simulink model "sim4el17128"  (R2019b)
settings: Solver=VariableStepAuto  StartTime=0.0  StopTime=20  RelTol=1e-4
values from neighbouring files (symbols this model uses):
  b1 = 0.0886    [sim_cm.m]    (also in sim_cm_LM_overestimate.m; sim_cm_LM_underestimate.m; sim_cm_RR_overestimate.m; sim_cm_RR_underestimate.m)
  b2 = 0.0012    [sim_cm.m]    (also in sim_cm_LM_overestimate.m; sim_cm_LM_underestimate.m; sim_cm_RR_overestimate.m; sim_cm_RR_underestimate.m)
  ba = (2*K^2*(alphaS*J-b1))/(3*np^2)    [sim_cm.m]    (also in sim_cm_LM_overestimate.m; sim_cm_LM_underestimate.m; sim_cm_RR_overestimate.m; sim_cm_RR_underestimate.m)
  Idref = psi_hat/LM_hat    (= 4.50282942603)    [sim_cm.m]    (also in sim_cm_LM_overestimate.m = 4.09348129639; sim_cm_LM_underestimate.m = 5.0031438067; sim_cm_RR_overestimate.m; sim_cm_RR_underestimate.m)
  Imax = 12    [sim_cm.m]    (also in sim_cm_LM_overestimate.m; sim_cm_LM_underestimate.m; sim_cm_RR_overestimate.m; sim_cm_RR_underestimate.m = 15)
  Iqref = sqrt(Iref^2-Idref^2)    [sim_cm.m]    (also in sim_cm_LM_overestimate.m; sim_cm_LM_underestimate.m; sim_cm_RR_overestimate.m; sim_cm_RR_underestimate.m)
  J = 0.08    [sim_cm.m]    (also in sim_cm_LM_overestimate.m; sim_cm_LM_underestimate.m; sim_cm_RR_overestimate.m; sim_cm_RR_underestimate.m)
  K = 1/sqrt(2)    [sim_cm.m]    (also in sim_cm_LM_overestimate.m; sim_cm_LM_underestimate.m; sim_cm_RR_overestimate.m; sim_cm_RR_underestimate.m)
  Ki = alphaC*(R+Ra)    [sim_cm.m]    (also in sim_cm_LM_overestimate.m; sim_cm_LM_underestimate.m; sim_cm_RR_overestimate.m; sim_cm_RR_underestimate.m)
  kip = alphaP*alphaP/psi_hat    (= 21723.518851)    [sim_cm.m]    (also in sim_cm_LM_overestimate.m; sim_cm_LM_underestimate.m; sim_cm_RR_overestimate.m; sim_cm_RR_underestimate.m)
  Kis = Kps*alphaS    [sim_cm.m]    (also in sim_cm_LM_overestimate.m; sim_cm_LM_underestimate.m; sim_cm_RR_overestimate.m; sim_cm_RR_underestimate.m)
  Kp = alphaC*L    [sim_cm.m]    (also in sim_cm_LM_overestimate.m; sim_cm_LM_underestimate.m; sim_cm_RR_overestimate.m; sim_cm_RR_underestimate.m)
  kpp = 2*alphaP/psi_hat    (= 394.973070018)    [sim_cm.m]    (also in sim_cm_LM_overestimate.m; sim_cm_LM_underestimate.m; sim_cm_RR_overestimate.m; sim_cm_RR_underestimate.m)
  Kps = (2*K^2*alphaS*J)/(3*np^2)    [sim_cm.m]    (also in sim_cm_LM_overestimate.m; sim_cm_LM_underestimate.m; sim_cm_RR_overestimate.m; sim_cm_RR_underestimate.m)
  L = Lsigma_hat    (= 0.0227)    [sim_cm.m]    (also in sim_cm_LM_overestimate.m; sim_cm_LM_underestimate.m; sim_cm_RR_overestimate.m; sim_cm_RR_underestimate.m)
  lamda = 2    [sim_cm.m]    (also in sim_cm_LM_overestimate.m; sim_cm_LM_underestimate.m; sim_cm_RR_overestimate.m; sim_cm_RR_underestimate.m)
  LM = 0.1237    [sim_cm.m]    (also in sim_cm_LM_overestimate.m; sim_cm_LM_underestimate.m; sim_cm_RR_overestimate.m; sim_cm_RR_underestimate.m)
  LM_hat = LM    (= 0.1237)    [sim_cm.m]    (also in sim_cm_LM_overestimate.m = 0.13607; sim_cm_LM_underestimate.m = 0.11133; sim_cm_RR_overestimate.m; sim_cm_RR_underestimate.m)
  Lsigma = 0.0227    [sim_cm.m]    (also in sim_cm_LM_overestimate.m; sim_cm_LM_underestimate.m; sim_cm_RR_overestimate.m; sim_cm_RR_underestimate.m)
  Lsigma_hat = Lsigma    (= 0.0227)    [sim_cm.m]    (also in sim_cm_LM_overestimate.m; sim_cm_LM_underestimate.m; sim_cm_RR_overestimate.m; sim_cm_RR_underestimate.m)
  np = 2    [sim_cm.m]    (also in sim_cm_LM_overestimate.m; sim_cm_LM_underestimate.m; sim_cm_RR_overestimate.m; sim_cm_RR_underestimate.m)
  phi_a = 0    [sim_cm.m]    (also in sim_cm_LM_overestimate.m; sim_cm_LM_underestimate.m; sim_cm_RR_overestimate.m; sim_cm_RR_underestimate.m)
  phi_b = -2*pi/3    (= -2.09439510239)    [sim_cm.m]    (also in sim_cm_LM_overestimate.m; sim_cm_LM_underestimate.m; sim_cm_RR_overestimate.m; sim_cm_RR_underestimate.m)
  phi_c = -4*pi/3    (= -4.18879020479)    [sim_cm.m]    (also in sim_cm_LM_overestimate.m; sim_cm_LM_underestimate.m; sim_cm_RR_overestimate.m; sim_cm_RR_underestimate.m)
  Ra = alphaC*L - R    [sim_cm.m]    (also in sim_cm_LM_overestimate.m; sim_cm_LM_underestimate.m; sim_cm_RR_overestimate.m; sim_cm_RR_underestimate.m)
  RR = 0.8197    [sim_cm.m]    (also in sim_cm_LM_overestimate.m; sim_cm_LM_underestimate.m; sim_cm_RR_overestimate.m; sim_cm_RR_underestimate.m)
  RR_hat = RR    (= 0.8197)    [sim_cm.m]    (also in sim_cm_LM_overestimate.m; sim_cm_LM_underestimate.m; sim_cm_RR_overestimate.m = 1.14758; sim_cm_RR_underestimate.m = 0.49182)
  Rs = 2.2667    [sim_cm.m]    (also in sim_cm_LM_overestimate.m; sim_cm_LM_underestimate.m; sim_cm_RR_overestimate.m; sim_cm_RR_underestimate.m)
  Rs_hat = Rs    (= 2.2667)    [sim_cm.m]    (also in sim_cm_LM_overestimate.m; sim_cm_LM_underestimate.m; sim_cm_RR_overestimate.m; sim_cm_RR_underestimate.m)
  sw1 = 1    [sim_cm.m]    (also in sim_cm_LM_overestimate.m; sim_cm_LM_underestimate.m; sim_cm_RR_overestimate.m; sim_cm_RR_underestimate.m)
  sw3 = 1    [sim_cm.m]    (also in sim_cm_LM_overestimate.m; sim_cm_LM_underestimate.m; sim_cm_RR_overestimate.m; sim_cm_RR_underestimate.m)
  sw4 = 1    [sim_cm.m]    (also in sim_cm_LM_overestimate.m; sim_cm_LM_underestimate.m; sim_cm_RR_overestimate.m; sim_cm_RR_underestimate.m)
  sw5 = 0    [sim_cm.m]    (also in sim_cm_LM_overestimate.m = 1; sim_cm_LM_underestimate.m = 1; sim_cm_RR_overestimate.m = 1; sim_cm_RR_underestimate.m = 1)
  sw6 = 0    [sim_cm.m]    (also in sim_cm_LM_overestimate.m; sim_cm_LM_underestimate.m; sim_cm_RR_overestimate.m; sim_cm_RR_underestimate.m)
  sw7 = 0    [sim_cm.m]    (also in sim_cm_LM_overestimate.m; sim_cm_LM_underestimate.m; sim_cm_RR_overestimate.m; sim_cm_RR_underestimate.m)
  tL = 26.8    [sim_cm.m]    (also in sim_cm_LM_overestimate.m; sim_cm_LM_underestimate.m; sim_cm_RR_overestimate.m; sim_cm_RR_underestimate.m)
  Un = 230    [sim_cm.m]    (also in sim_cm_LM_overestimate.m; sim_cm_LM_underestimate.m; sim_cm_RR_overestimate.m; sim_cm_RR_underestimate.m)
  Vhat = 230*sqrt(2)    [sim_cm.m]    (also in sim_cm_LM_overestimate.m; sim_cm_LM_underestimate.m; sim_cm_RR_overestimate.m; sim_cm_RR_underestimate.m)
  w = 2*pi*f    (= 314.159265359)    [sim_cm.m]    (also in sim_cm_LM_overestimate.m; sim_cm_LM_underestimate.m; sim_cm_RR_overestimate.m; sim_cm_RR_underestimate.m)
  wdelta = 0.2*wbase    (= 60.48)    [sim_cm.m]    (also in sim_cm_LM_overestimate.m; sim_cm_LM_underestimate.m; sim_cm_RR_overestimate.m; sim_cm_RR_underestimate.m)
undefined symbols (not defined in the file or in its folder): magnitude, sigbuilder_block
libraries: simulink x1
settings Model: DataTypeOverride=Double  MinMaxOverflowLogging=ForceOff  Creator=user  LastModifiedBy=user
settings SolverCC: ZeroCrossAlgorithm=Adaptive
settings DebuggingCC: IgnoredZcDiagnostic=none

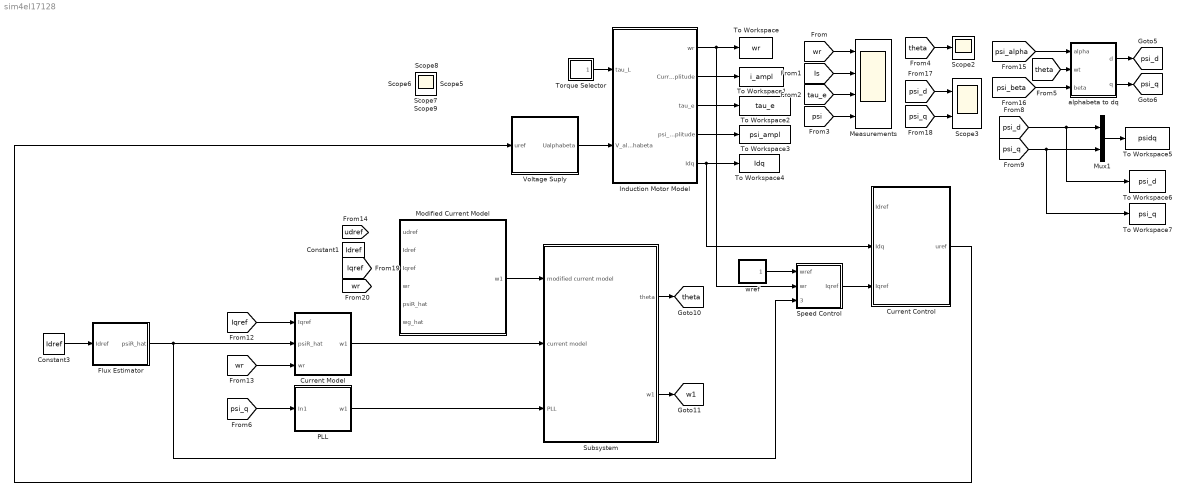
== system sim4el17128 ==
  Constant1 : Constant  Value=Idref
  Constant3 : Constant  Value=Idref
  Current Control : Subsystem
  Current Model : Subsystem
  Flux Estimator : Subsystem
  Induction Motor Model : Subsystem
  Measurements : Scope  NumInputPorts=4
  Modified Current Model : Subsystem
  Mux1 : Mux  Inputs=2
  PLL : Subsystem
  Scope{,1..2,4..9} (9 alike) : Scope
  Scope3 : Scope  NumInputPorts=2
  Speed Control : Subsystem
  Subsystem : Subsystem
  To Workspace : ToWorkspace  VariableName=wr  SaveFormat=Timeseries  SampleTime=-1
  To Workspace1 : ToWorkspace  VariableName=i_ampl  SaveFormat=Timeseries  SampleTime=-1
  To Workspace2 : ToWorkspace  VariableName=tau_e  SaveFormat=Timeseries  SampleTime=-1
  To Workspace3 : ToWorkspace  VariableName=psi_ampl  SaveFormat=Timeseries  SampleTime=-1
  To Workspace4 : ToWorkspace  VariableName=Idq  SaveFormat=Timeseries  SampleTime=-1
  To Workspace5 : ToWorkspace  VariableName=psidq  SaveFormat=Timeseries  SampleTime=-1
  To Workspace6 : ToWorkspace  VariableName=psi_d  SaveFormat=Timeseries  SampleTime=-1
  To Workspace7 : ToWorkspace  VariableName=psi_q  SaveFormat=Timeseries  SampleTime=-1
  Torque Selector : Subsystem
  Voltage Suply : Subsystem
  alphabeta to dq : Subsystem
  wref : Subsystem
  tag scope: psi_d=global, psi_q=global, theta=global, w1=global
  wires:
  Induction Motor Model/1(wr) -> Speed Control/2(wr), To Workspace/1
  Induction Motor Model/3(tau_e) -> To Workspace2/1
  Induction Motor Model/2(Current amplitude) -> To Workspace1/1
  Induction Motor Model/4(psi_amplitude) -> To Workspace3/1
  [wr] -> Measurements/1
  [Is] -> Measurements/2
  [tau_e] -> Measurements/3
  [psi] -> Measurements/4
  [theta] -> Scope2/1
  [psi_q] -> Scope3/2
  [psi_d] -> Scope3/1
  alphabeta to dq/2(q) -> [psi_q]
  [psi_alpha] -> alphabeta to dq/1(alpha)
  [psi_beta] -> alphabeta to dq/3(beta)
  alphabeta to dq/1(d) -> [psi_d]
  Induction Motor Model/5(Idq) -> To Workspace4/1, Current Control/2(Idq)
  Torque Selector/1(tau_L) -> Induction Motor Model/1(tau_L)
  [psi_q] -> To Workspace7/1, Mux1/2
  [psi_d] -> To Workspace6/1, Mux1/1
  Mux1/1 -> To Workspace5/1
  Current Control/1(uref) -> Voltage Suply/1(uref)
  Voltage Suply/1(Ualphabeta) -> Induction Motor Model/2(V_alphabeta)
  Speed Control/1(Iqref) -> Current Control/3(Iqref)
  wref/1(Out1) -> Speed Control/1(wref)
  [theta] -> alphabeta to dq/2(wt)
  Subsystem/1(theta) -> [theta]
  Subsystem/2(w1) -> [w1]
  [Iqref] -> Current Model/1(Iqref)
  [wr] -> Current Model/3(wr)
  [psi_q] -> PLL/1(In1)
  Current Model/1(w1) -> Subsystem/2(current model)
  PLL/1(w1) -> Subsystem/3(PLL)
  Constant3/1 -> Flux Estimator/1(Idref)
  Flux Estimator/1(psiR_hat) -> Speed Control/3(psiR_hat), Current Model/2(psiR_hat)
  Modified Current Model/1(w1) -> Subsystem/1(modified current model)

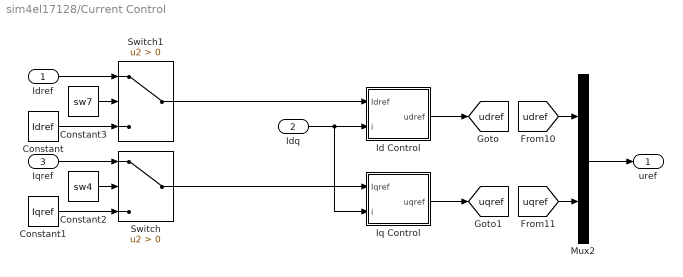
== system sim4el17128/Current Control ==
  Idref : Inport
  Idq : Inport  Port=2
  Iqref : Inport  Port=3
  Constant : Constant  Value=Idref
  Constant1 : Constant  Value=Iqref
  Constant2 : Constant  Value=sw4
  Constant3 : Constant  Value=sw7
  Id Control : Subsystem
  Iq Control : Subsystem
  Mux2 : Mux  Inputs=2
  Switch : Switch  Criteria=u2 > Threshold
  Switch1 : Switch  Criteria=u2 > Threshold
  uref : Outport
  tag scope: udref=global, uqref=global
  wires:
  [uqref] -> Mux2/2
  Iq Control/1(uqref) -> [uqref]
  Idq/1 -> Id Control/2(i), Iq Control/2(i)
  Mux2/1 -> uref/1
  [udref] -> Mux2/1
  Id Control/1(udref) -> [udref]
  Iqref/1 -> Switch/1
  Switch/1 -> Iq Control/1(Iqref)
  Constant2/1 -> Switch/2
  Constant1/1 -> Switch/3
  Switch1/1 -> Id Control/1(Idref)
  Constant/1 -> Switch1/3
  Constant3/1 -> Switch1/2
  Idref/1 -> Switch1/1

== system sim4el17128/Current Model ==
  Iqref : Inport
  psiR_hat : Inport  Port=2
  wr : Inport  Port=3
  Gain : Gain  Gain=RR_hat
  Product : Product  Inputs=*/
  Sum : Sum
  w1 : Outport
  wires:
  wr/1 -> Sum/2
  Sum/1 -> w1/1
  Iqref/1 -> Gain/1
  Gain/1 -> Product/1
  Product/1 -> Sum/1
  psiR_hat/1 -> Product/2

== system sim4el17128/Flux Estimator ==
  Idref : Inport
  Clock : Clock
  Constant4 : Constant  Value=0.001
  Gain : Gain  Gain=RR_hat
  Gain1 : Gain  Gain=1/LM_hat
  Integrator : Integrator
  Sum : Sum  Inputs=|+-
  Switch : Switch  Criteria=u2 > Threshold  Threshold=0.001
  psiR_hat : Outport
  wires:
  Clock/1 -> Switch/2
  Constant4/1 -> Switch/3
  Integrator/1 -> Gain1/1, Switch/1
  Gain1/1 -> Sum/2
  Sum/1 -> Gain/1
  Gain/1 -> Integrator/1
  Idref/1 -> Sum/1
  Switch/1 -> psiR_hat/1

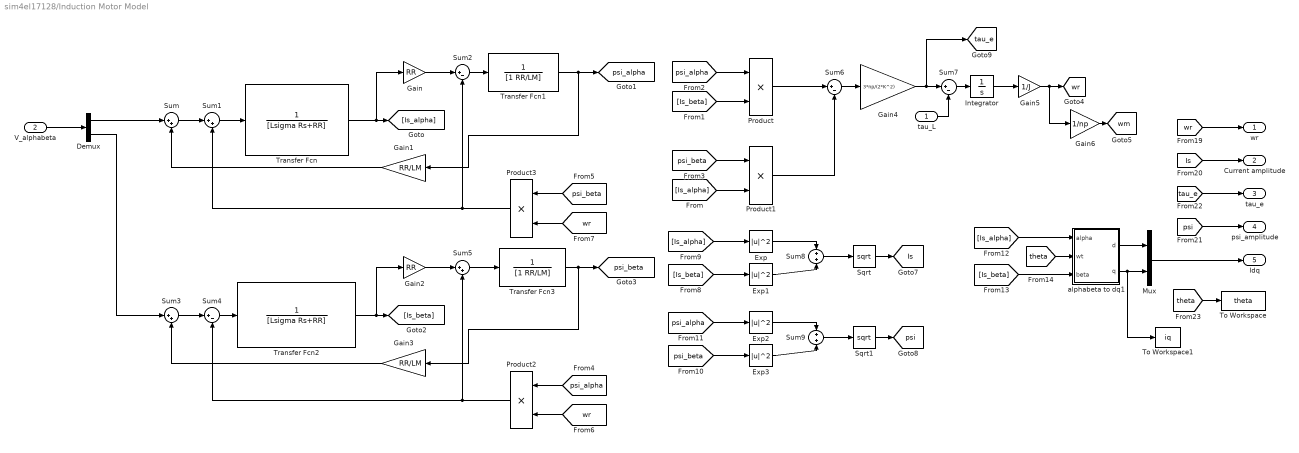
== system sim4el17128/Induction Motor Model ==
  tau_L : Inport
  V_alphabeta : Inport  Port=2
  Demux : Demux  Outputs=2
  Exp{,1..3} (4 alike) : Math  Operator=magnitude^2  SignedPower=off  SaturateOnIntegerOverflow=on
  Gain : Gain  Gain=RR
  Gain1 : Gain  Gain=RR/LM
  Gain2 : Gain  Gain=RR
  Gain3 : Gain  Gain=RR/LM
  Gain4 : Gain  Gain=3*np/(2*K^2)
  Gain5 : Gain  Gain=1/J
  Gain6 : Gain  Gain=1/np
  Integrator : Integrator
  Mux : Mux  Inputs=2
  Product{,1..3} (4 alike) : Product
  Sqrt : Sqrt  SaturateOnIntegerOverflow=on
  Sqrt1 : Sqrt  SaturateOnIntegerOverflow=on
  Sum{,1,3,5} (4 alike) : Sum  Inputs=|++
  Sum{2,4,6..7} (4 alike) : Sum  Inputs=|+-
  Sum8 : Sum  Inputs=+|+
  Sum9 : Sum  Inputs=+|+
  To Workspace : ToWorkspace  VariableName=theta  SaveFormat=Timeseries  SampleTime=-1
  To Workspace1 : ToWorkspace  VariableName=iq  SaveFormat=Timeseries  SampleTime=-1
  Transfer Fcn : TransferFcn  Denominator=[Lsigma Rs+RR]
  Transfer Fcn1 : TransferFcn  Denominator=[1 RR/LM]
  Transfer Fcn2 : TransferFcn  Denominator=[Lsigma Rs+RR]
  Transfer Fcn3 : TransferFcn  Denominator=[1 RR/LM]
  alphabeta to dq1 : Subsystem
  wr : Outport
  Current amplitude : Outport  Port=2
  tau_e : Outport  Port=3
  psi_amplitude : Outport  Port=4
  Idq : Outport  Port=5
  tag scope: Is=global, psi=global, psi_alpha=global, psi_beta=global, tau_e=global, wm=global, wr=global
  wires:
  Transfer Fcn1/1 -> Gain1/1, [psi_alpha]
  Product3/1 -> Sum1/2, Sum2/2
  Product2/1 -> Sum4/2, Sum5/2
  [Is_beta] -> Exp1/1
  Gain5/1 -> Gain6/1, [wr]
  [Is_beta] -> Product/2
  Product/1 -> Sum6/1
  [wr] -> Product2/2
  Sqrt/1 -> [Is]
  Sum3/1 -> Sum4/1
  Transfer Fcn3/1 -> Gain3/1, [psi_beta]
  [psi_beta] -> Product1/1
  Sum5/1 -> Transfer Fcn3/1
  Transfer Fcn2/1 -> Gain2/1, [Is_beta]
  Sum1/1 -> Transfer Fcn/1
  V_alphabeta/1 -> Demux/1
  [Is_alpha] -> Product1/2
  Gain1/1 -> Sum/2
  Demux/2 -> Sum3/1
  Demux/1 -> Sum/1
  Exp/1 -> Sum8/1
  tau_L/1 -> Sum7/2
  Sum/1 -> Sum1/1
  Sum6/1 -> Gain4/1
  Gain4/1 -> [tau_e], Sum7/1
  Transfer Fcn/1 -> Gain/1, [Is_alpha]
  [psi_alpha] -> Product/1
  Sum2/1 -> Transfer Fcn1/1
  Gain3/1 -> Sum3/2
  Gain2/1 -> Sum5/1
  Sum4/1 -> Transfer Fcn2/1
  Product1/1 -> Sum6/2
  [Is_alpha] -> Exp/1
  Sum8/1 -> Sqrt/1
  Gain/1 -> Sum2/1
  [wr] -> Product3/2
  [psi_beta] -> Product3/1
  Sum7/1 -> Integrator/1
  Integrator/1 -> Gain5/1
  [psi_alpha] -> Product2/1
  Exp1/1 -> Sum8/2
  Sum9/1 -> Sqrt1/1
  [psi_alpha] -> Exp2/1
  Exp3/1 -> Sum9/2
  [psi_beta] -> Exp3/1
  Exp2/1 -> Sum9/1
  Sqrt1/1 -> [psi]
  Mux/1 -> Idq/1
  alphabeta to dq1/2(q) -> To Workspace1/1, Mux/2
  alphabeta to dq1/1(d) -> Mux/1
  [Is_beta] -> alphabeta to dq1/3(beta)
  [Is_alpha] -> alphabeta to dq1/1(alpha)
  [theta] -> alphabeta to dq1/2(wt)
  [wr] -> wr/1
  [Is] -> Current amplitude/1
  [psi] -> psi_amplitude/1
  [tau_e] -> tau_e/1
  [theta] -> To Workspace/1
  Gain6/1 -> [wm]

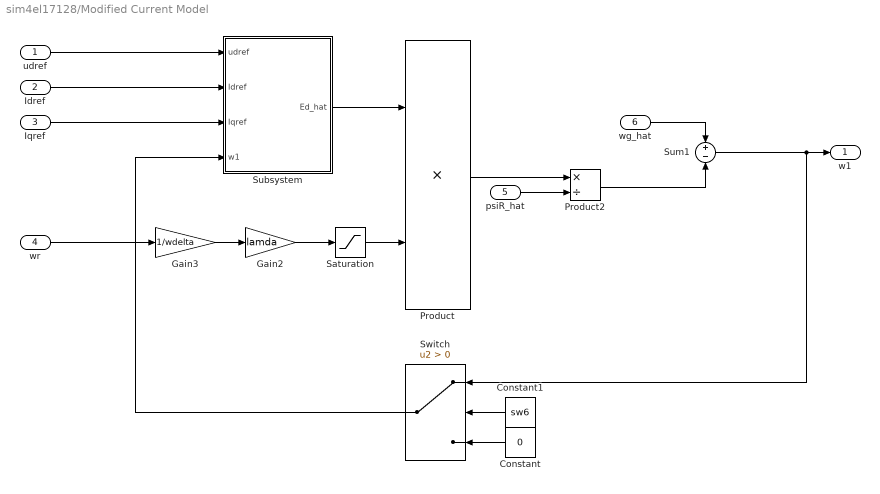
== system sim4el17128/Modified Current Model ==
  udref : Inport
  Idref : Inport  Port=2
  Iqref : Inport  Port=3
  wr : Inport  Port=4
  psiR_hat : Inport  Port=5
  wg_hat : Inport  Port=6
  Constant : Constant  Value=0
  Constant1 : Constant  Value=sw6
  Gain2 : Gain  Gain=lamda
  Gain3 : Gain  Gain=1/wdelta
  Product : Product
  Product2 : Product  Inputs=*/
  Saturation : Saturate  UpperLimit=lamda  LowerLimit=-lamda
  Subsystem : Subsystem
  Sum1 : Sum  Inputs=+-
  Switch : Switch  Criteria=u2 > Threshold
  w1 : Outport
  wires:
  Sum1/1 -> Switch/1, w1/1
  Product/1 -> Product2/1
  Switch/1 -> Subsystem/4(w1)
  Constant/1 -> Switch/3
  Constant1/1 -> Switch/2
  Idref/1 -> Subsystem/2(Idref)
  udref/1 -> Subsystem/1(udref)
  Subsystem/1(Ed_hat) -> Product/1
  Gain3/1 -> Gain2/1
  Gain2/1 -> Saturation/1
  Saturation/1 -> Product/2
  Iqref/1 -> Subsystem/3(Iqref)
  wr/1 -> Gain3/1
  psiR_hat/1 -> Product2/2
  Product2/1 -> Sum1/2
  wg_hat/1 -> Sum1/1

== system sim4el17128/PLL ==
  In1 : Inport
  Gain8 : Gain  Gain=kpp
  Gain9 : Gain  Gain=kip
  Integrator1 : Integrator
  Sum13 : Sum  Inputs=+++
  wg : Constant  Value=w
  w1 : Outport
  wires:
  In1/1 -> Gain9/1, Gain8/1  "ψq"
  Gain8/1 -> Sum13/2
  wg/1 -> Sum13/1
  Gain9/1 -> Integrator1/1
  Integrator1/1 -> Sum13/3
  Sum13/1 -> w1/1

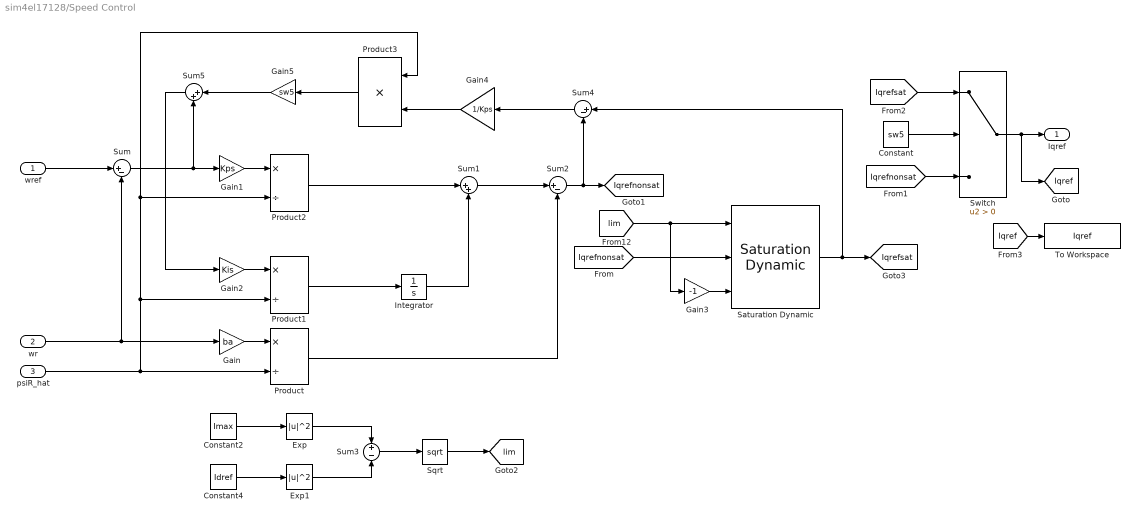
== system sim4el17128/Speed Control ==
  wref : Inport
  wr : Inport  Port=2
  psiR_hat : Inport  Port=3
  Constant : Constant  Value=sw5
  Constant2 : Constant  Value=Imax
  Constant4 : Constant  Value=Idref
  Exp : Math  Operator=magnitude^2  SignedPower=off  SaturateOnIntegerOverflow=on
  Exp1 : Math  Operator=magnitude^2  SignedPower=off  SaturateOnIntegerOverflow=on
  Gain : Gain  Gain=ba
  Gain1 : Gain  Gain=Kps
  Gain2 : Gain  Gain=Kis
  Gain3 : Gain  Gain=-1
  Gain4 : Gain  Gain=1/Kps
  Gain5 : Gain  Gain=sw5
  Integrator : Integrator
  Product : Product  Inputs=*/
  Product1 : Product  Inputs=*/
  Product2 : Product  Inputs=*/
  Product3 : Product
  Saturation Dynamic : simulink/Discontinuities/Saturation Dynamic  OutMin=[]  OutMax=[]  OutDataTypeStr=Inherit: Same as second input  OutDataType=fixdt(1, 16)  OutScaling=2^-10  DoSatur=off
  Sqrt : Sqrt  SaturateOnIntegerOverflow=on
  Sum : Sum  Inputs=|+-
  Sum1 : Sum  Inputs=|++
  Sum2 : Sum  Inputs=|+-
  Sum3 : Sum  Inputs=+-
  Sum4 : Sum  Inputs=|+-
  Sum5 : Sum  Inputs=|++
  Switch : Switch  Criteria=u2 > Threshold
  To Workspace : ToWorkspace  VariableName=Iqref  SaveFormat=Timeseries  SampleTime=-1
  Iqref : Outport
  tag scope: Iqref=global, Iqrefnonsat=global, Iqrefsat=global, lim=global
  wires:
  Sum3/1 -> Sqrt/1
  Exp/1 -> Sum3/1
  Sum/1 -> Sum5/2, Gain1/1
  Gain3/1 -> Saturation Dynamic/3
  wr/1 -> Sum/2, Gain/1
  Constant4/1 -> Exp1/1
  Exp1/1 -> Sum3/2
  Sum1/1 -> Sum2/1
  Sum4/1 -> Gain4/1
  Integrator/1 -> Sum1/2
  wref/1 -> Sum/1
  Gain5/1 -> Sum5/1
  [lim] -> Gain3/1, Saturation Dynamic/1
  Sum2/1 -> Sum4/2, [Iqrefnonsat]
  [Iqrefnonsat] -> Saturation Dynamic/2
  Saturation Dynamic/1 -> [Iqrefsat], Sum4/1
  [Iqrefnonsat] -> Switch/3
  Switch/1 -> Iqref/1, [Iqref]
  [Iqrefsat] -> Switch/1
  Constant/1 -> Switch/2
  Sum5/1 -> Gain2/1
  Sqrt/1 -> [lim]
  Gain/1 -> Product/1
  Product/1 -> Sum2/2
  Constant2/1 -> Exp/1
  psiR_hat/1 -> Product/2, Product1/2, Product2/2, Product3/1
  Gain2/1 -> Product1/1
  Product1/1 -> Integrator/1
  Gain1/1 -> Product2/1
  Product2/1 -> Sum1/1
  Product3/1 -> Gain5/1
  Gain4/1 -> Product3/2
  [Iqref] -> To Workspace/1

== system sim4el17128/Subsystem ==
  modified current model : Inport
  current model : Inport  Port=2
  PLL : Inport  Port=3
  Constant : Constant  Value=sw4
  Constant1 : Constant  Value=sw6
  Constant2 : Constant  Value=sw7
  Constant5 : Constant  Value=2*pi
  Integrator2 : Integrator
  Mod : Math  Operator=mod  SignedPower=off  SaturateOnIntegerOverflow=on
  Switch : Switch  Criteria=u2 > Threshold
  Switch1 : Switch  Criteria=u2 > Threshold
  Switch2 : Switch  Criteria=u2 > Threshold
  theta : Outport
  w1 : Outport  Port=2
  wires:
  modified current model/1 -> Switch1/1
  Constant/1 -> Switch/2
  Constant1/1 -> Switch1/2
  Switch/1 -> Switch1/3
  current model/1 -> Switch/1
  PLL/1 -> Switch/3
  Mod/1 -> theta/1
  Constant5/1 -> Mod/2
  Integrator2/1 -> Mod/1
  Switch1/1 -> Switch2/3
  Switch2/1 -> w1/1, Integrator2/1
  Constant2/1 -> Switch2/2

== system sim4el17128/Torque Selector ==
  Constant : Constant  Value=0
  Exp : Math  Operator=magnitude^2  SignedPower=off  SaturateOnIntegerOverflow=on
  Gain : Gain  Gain=b1
  Gain1 : Gain  Gain=b2
  Manual Switch : ManualSwitch  CurrentSetting=0
  Manual Switch1 : ManualSwitch
  Manual Switch2 : ManualSwitch  CurrentSetting=0
  taul_L : Step  Time=5  After=tL  SampleTime=0
  tau_L : Outport
  wires:
  [wr] -> Gain/1
  Gain1/1 -> Manual Switch1/2
  taul_L/1 -> Manual Switch/2
  Exp/1 -> Gain1/1
  [wm] -> Exp/1
  Constant/1 -> Manual Switch/1
  Gain/1 -> Manual Switch1/1
  Manual Switch2/1 -> tau_L/1
  Manual Switch1/1 -> Manual Switch2/2
  Manual Switch/1 -> Manual Switch2/1

== system sim4el17128/Voltage Suply ==
  uref : Inport
  Constant2 : Constant  Value=sw1
  Demux : Demux  Outputs=2
  Grid Voltage : Subsystem
  Mux : Mux  Inputs=2
  Scope1 : Scope
  Switch : Switch  Criteria=u2 > Threshold
  dq to alphabeta : Subsystem
  Ualphabeta : Outport
  wires:
  Grid Voltage/2(V_dq) -> Scope1/1
  Constant2/1 -> Switch/2
  Mux/1 -> Switch/1
  Demux/2 -> dq to alphabeta/3(q)
  Demux/1 -> dq to alphabeta/1(d)
  Grid Voltage/1(V_alphabeta) -> Switch/3
  [theta] -> dq to alphabeta/2(wt)
  dq to alphabeta/1(alpha) -> Mux/1
  dq to alphabeta/2(beta) -> Mux/2
  uref/1 -> Demux/1
  Switch/1 -> Ualphabeta/1  "Ualphabeta"

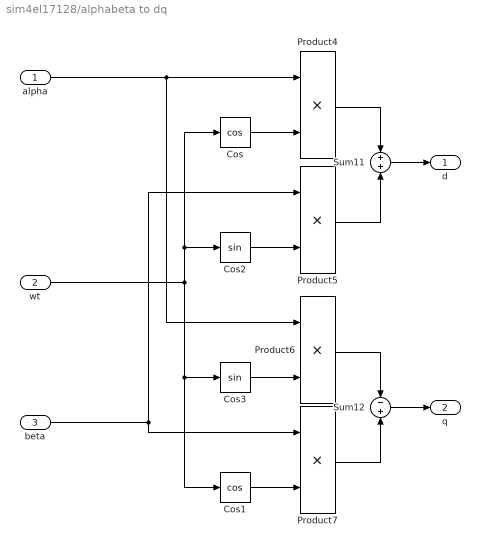
== system sim4el17128/alphabeta to dq ==
  alpha : Inport
  wt : Inport  Port=2
  beta : Inport  Port=3
  Cos : Trigonometry  Operator=cos
  Cos1 : Trigonometry  Operator=cos
  Cos2 : Trigonometry
  Cos3 : Trigonometry
  Product{4..7} (4 alike) : Product
  Sum11 : Sum
  Sum12 : Sum  Inputs=-+
  d : Outport
  q : Outport  Port=2
  wires:
  Cos3/1 -> Product6/2
  Product6/1 -> Sum12/1
  Sum11/1 -> d/1
  alpha/1 -> Product4/1, Product6/1
  wt/1 -> Cos3/1, Cos1/1, Cos2/1, Cos/1
  Product4/1 -> Sum11/1
  beta/1 -> Product7/1, Product5/1
  Product7/1 -> Sum12/2
  Cos1/1 -> Product7/2
  Product5/1 -> Sum11/2
  Cos/1 -> Product4/2
  Cos2/1 -> Product5/2
  Sum12/1 -> q/1

== system sim4el17128/wref ==
  Constant : Constant  Value=sw7
  Manual Switch : ManualSwitch
  Signal Builder : Subsystem  Tag=STV Subsys  LoadFcn=sigbuilder_block('load');  StartFcn=sigbuilder_block('start');  StopFcn=sigbuilder_block('stop');  ClipboardFcn=sigbuilder_block('clipboard');  mask(Sigbuilder block){tuvar=[0:10]}
      mask help: Simulink:masks:SigbuilderBlock_MD
      mask init:
      | if ~strcmp(get_param(bdroot(gcbh),'SimulationStatus'),'stopped') tuvar = sigbuilder_block('maskInit'); end
      settings: CopyFcn=sigbuilder_block('copy');  DeleteFcn=sigbuilder_block('delete');  ModelCloseFcn=sigbuilder_block('modelClose');  PreSaveFcn=sigbuilder_block('preSave');  PauseFcn=sigbuilder_block('pause');  ContinueFcn=sigbuilder_block('continue');  NameChangeFcn=sigbuilder_block('namechange');  OpenFcn=sigbuilder_block('open',[6 30 1012.5 447.75 ]);  CloseFcn=sigbuilder_block('close');
      mask Display: plot(0, 0, 100, 100,[2, 2, 32, 32, 2], [68, 8, 8, 68, 68],[32, 2], [38, 38], [32, 19, 2],[53, 60, 44], [32, 17, 17, 2],[16, 16, 31, 31]);txt = getActiveGroup(gcbh);text(2, 100, txt,'verticalAlignment', 'top');
  Switch : Switch  Criteria=u2 > Threshold
  To Workspace : ToWorkspace  VariableName=wref  SaveFormat=Timeseries  SampleTime=-1
  Out1 : Outport
  wires:
  Signal Builder/2(wrefnom) -> Manual Switch/2
  Signal Builder/1(wref) -> Manual Switch/1
  Manual Switch/1 -> Switch/3
  Signal Builder/3(field weakening) -> Switch/1
  Switch/1 -> To Workspace/1, Out1/1
  Constant/1 -> Switch/2

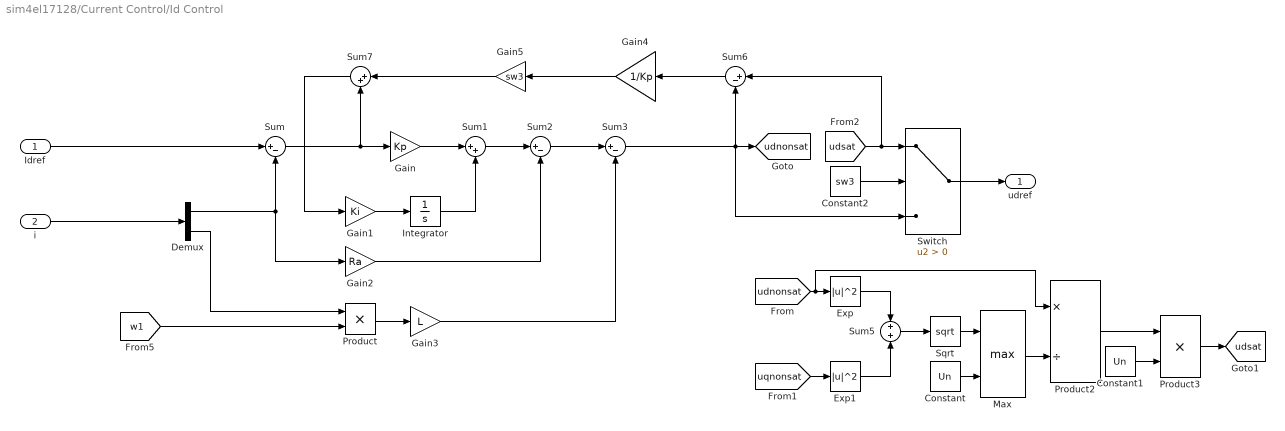
== system sim4el17128/Current Control/Id Control ==
  Idref : Inport
  i : Inport  Port=2
  Constant : Constant  Value=Un
  Constant1 : Constant  Value=Un
  Constant2 : Constant  Value=sw3
  Demux : Demux  Outputs=2
  Exp : Math  Operator=magnitude^2  SignedPower=off  SaturateOnIntegerOverflow=on
  Exp1 : Math  Operator=magnitude^2  SignedPower=off  SaturateOnIntegerOverflow=on
  Gain : Gain  Gain=Kp
  Gain1 : Gain  Gain=Ki
  Gain2 : Gain  Gain=Ra
  Gain3 : Gain  Gain=L
  Gain4 : Gain  Gain=1/Kp
  Gain5 : Gain  Gain=sw3
  Integrator : Integrator
  Max : MinMax  Function=max  Inputs=2
  Product : Product
  Product2 : Product  Inputs=*/
  Product3 : Product
  Sqrt : Sqrt  SaturateOnIntegerOverflow=on
  Sum{,2..3,6} (4 alike) : Sum  Inputs=|+-
  Sum1 : Sum  Inputs=|++
  Sum5 : Sum
  Sum7 : Sum  Inputs=|++
  Switch : Switch  Criteria=u2 > Threshold
  udref : Outport
  tag scope: udnonsat=global, udsat=global
  wires:
  Sum/1 -> Sum7/2, Gain/1
  Demux/2 -> Product/1
  Gain2/1 -> Sum2/2
  Demux/1 -> Gain2/1, Sum/2
  Gain/1 -> Sum1/1
  Sum2/1 -> Sum3/1
  Sum1/1 -> Sum2/1
  Gain1/1 -> Integrator/1
  Product/1 -> Gain3/1
  Integrator/1 -> Sum1/2
  i/1 -> Demux/1
  Idref/1 -> Sum/1
  [udnonsat] -> Product2/1, Exp/1
  [uqnonsat] -> Exp1/1
  Exp/1 -> Sum5/1
  Exp1/1 -> Sum5/2
  Sum5/1 -> Sqrt/1
  Sqrt/1 -> Max/1
  Constant/1 -> Max/2
  Max/1 -> Product2/2
  Product2/1 -> Product3/1
  Constant1/1 -> Product3/2
  Product3/1 -> [udsat]
  [udsat] -> Switch/1, Sum6/1
  Sum7/1 -> Gain1/1
  Gain4/1 -> Gain5/1
  Sum6/1 -> Gain4/1
  [w1] -> Product/2
  Switch/1 -> udref/1
  Constant2/1 -> Switch/2
  Gain5/1 -> Sum7/1
  Gain3/1 -> Sum3/2
  Sum3/1 -> Switch/3, Sum6/2, [udnonsat]

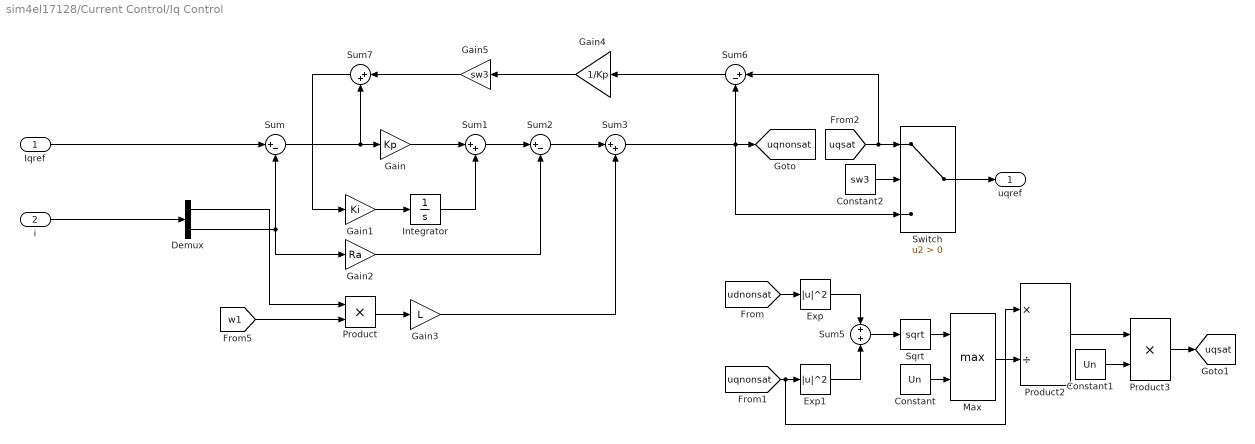
== system sim4el17128/Current Control/Iq Control ==
  Iqref : Inport
  i : Inport  Port=2
  Constant : Constant  Value=Un
  Constant1 : Constant  Value=Un
  Constant2 : Constant  Value=sw3
  Demux : Demux  Outputs=2
  Exp : Math  Operator=magnitude^2  SignedPower=off  SaturateOnIntegerOverflow=on
  Exp1 : Math  Operator=magnitude^2  SignedPower=off  SaturateOnIntegerOverflow=on
  Gain : Gain  Gain=Kp
  Gain1 : Gain  Gain=Ki
  Gain2 : Gain  Gain=Ra
  Gain3 : Gain  Gain=L
  Gain4 : Gain  Gain=1/Kp
  Gain5 : Gain  Gain=sw3
  Integrator : Integrator
  Max : MinMax  Function=max  Inputs=2
  Product : Product
  Product2 : Product  Inputs=*/
  Product3 : Product
  Sqrt : Sqrt  SaturateOnIntegerOverflow=on
  Sum : Sum  Inputs=|+-
  Sum1 : Sum  Inputs=|++
  Sum2 : Sum  Inputs=|+-
  Sum3 : Sum  Inputs=|++
  Sum5 : Sum
  Sum6 : Sum  Inputs=|+-
  Sum7 : Sum  Inputs=|++
  Switch : Switch  Criteria=u2 > Threshold
  uqref : Outport
  tag scope: uqnonsat=global, uqsat=global
  wires:
  Iqref/1 -> Sum/1
  i/1 -> Demux/1
  Integrator/1 -> Sum1/2
  Product/1 -> Gain3/1
  Gain1/1 -> Integrator/1
  Sum1/1 -> Sum2/1
  Sum2/1 -> Sum3/1
  Gain/1 -> Sum1/1
  Gain2/1 -> Sum2/2
  [w1] -> Product/2
  Demux/2 -> Sum/2, Gain2/1
  Demux/1 -> Product/1
  Sum/1 -> Sum7/2, Gain/1
  Exp1/1 -> Sum5/2
  Constant1/1 -> Product3/2
  Max/1 -> Product2/2
  Sum5/1 -> Sqrt/1
  Constant/1 -> Max/2
  Product3/1 -> [uqsat]
  Sqrt/1 -> Max/1
  Product2/1 -> Product3/1
  [uqnonsat] -> Product2/1, Exp1/1
  Exp/1 -> Sum5/1
  [udnonsat] -> Exp/1
  Sum6/1 -> Gain4/1
  Gain4/1 -> Gain5/1
  Sum7/1 -> Gain1/1
  [uqsat] -> Sum6/1, Switch/1
  Switch/1 -> uqref/1
  Constant2/1 -> Switch/2
  Gain5/1 -> Sum7/1
  Sum3/1 -> Switch/3, Sum6/2, [uqnonsat]
  Gain3/1 -> Sum3/2

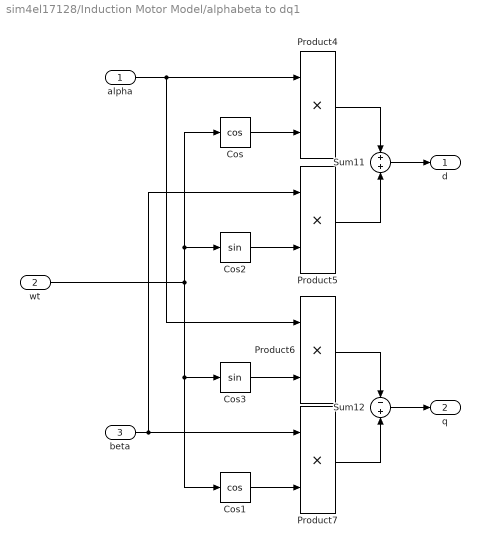
== system sim4el17128/Induction Motor Model/alphabeta to dq1 ==
  alpha : Inport
  wt : Inport  Port=2
  beta : Inport  Port=3
  Cos : Trigonometry  Operator=cos
  Cos1 : Trigonometry  Operator=cos
  Cos2 : Trigonometry
  Cos3 : Trigonometry
  Product{4..7} (4 alike) : Product
  Sum11 : Sum
  Sum12 : Sum  Inputs=-+
  d : Outport
  q : Outport  Port=2
  wires:
  Sum12/1 -> q/1
  Cos2/1 -> Product5/2
  Cos/1 -> Product4/2
  Product5/1 -> Sum11/2
  Cos1/1 -> Product7/2
  Product7/1 -> Sum12/2
  beta/1 -> Product7/1, Product5/1
  Product4/1 -> Sum11/1
  wt/1 -> Cos/1, Cos2/1, Cos1/1, Cos3/1
  alpha/1 -> Product6/1, Product4/1
  Sum11/1 -> d/1
  Product6/1 -> Sum12/1
  Cos3/1 -> Product6/2

== system sim4el17128/Modified Current Model/Subsystem ==
  udref : Inport
  Idref : Inport  Port=2
  Iqref : Inport  Port=3
  w1 : Inport  Port=4
  Gain : Gain  Gain=Rs_hat
  Gain1 : Gain  Gain=Lsigma_hat
  Product : Product
  Sum : Sum  Inputs=+-+
  Ed_hat : Outport
  wires:
  Sum/1 -> Ed_hat/1
  Iqref/1 -> Product/1
  udref/1 -> Sum/1
  Gain/1 -> Sum/2
  Idref/1 -> Gain/1
  Product/1 -> Gain1/1
  Gain1/1 -> Sum/3
  w1/1 -> Product/2

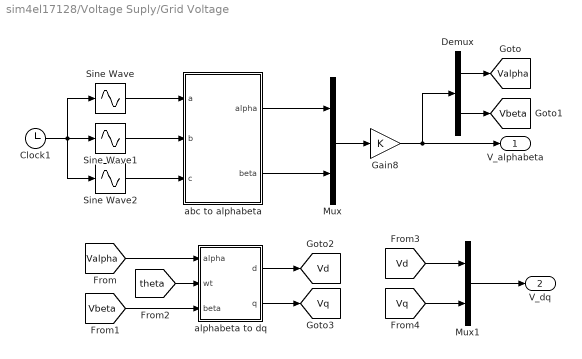
== system sim4el17128/Voltage Suply/Grid Voltage ==
  Clock1 : Clock
  Demux : Demux  Outputs=2
  Gain8 : Gain  Gain=K
  Mux : Mux  Inputs=2
  Mux1 : Mux  Inputs=2
  Sine Wave : Sin  TimeSource=Use external signal  Amplitude=Vhat  Frequency=w  Phase=phi_a  SampleTime=0
  Sine Wave1 : Sin  TimeSource=Use external signal  Amplitude=Vhat  Frequency=w  Phase=phi_b  SampleTime=0
  Sine Wave2 : Sin  TimeSource=Use external signal  Amplitude=Vhat  Frequency=w  Phase=phi_c  SampleTime=0
  abc to alphabeta : Subsystem
  alphabeta to dq : Subsystem
  V_alphabeta : Outport
  V_dq : Outport  Port=2
  tag scope: Valpha=global, Vbeta=global, Vd=global, Vq=global
  wires:
  Clock1/1 -> Sine Wave1/1, Sine Wave2/1, Sine Wave/1
  Mux/1 -> Gain8/1
  Gain8/1 -> Demux/1, V_alphabeta/1
  Demux/2 -> [Vbeta]
  Demux/1 -> [Valpha]
  [Valpha] -> alphabeta to dq/1(alpha)
  [Vbeta] -> alphabeta to dq/3(beta)
  [theta] -> alphabeta to dq/2(wt)
  alphabeta to dq/1(d) -> [Vd]
  alphabeta to dq/2(q) -> [Vq]
  [Vq] -> Mux1/2
  [Vd] -> Mux1/1
  Mux1/1 -> V_dq/1
  Sine Wave/1 -> abc to alphabeta/1(a)
  Sine Wave1/1 -> abc to alphabeta/2(b)
  Sine Wave2/1 -> abc to alphabeta/3(c)
  abc to alphabeta/1(alpha) -> Mux/1
  abc to alphabeta/2(beta) -> Mux/2

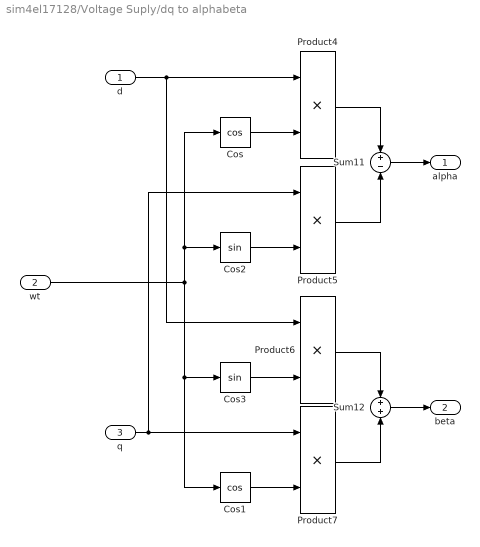
== system sim4el17128/Voltage Suply/dq to alphabeta ==
  d : Inport
  wt : Inport  Port=2
  q : Inport  Port=3
  Cos : Trigonometry  Operator=cos
  Cos1 : Trigonometry  Operator=cos
  Cos2 : Trigonometry
  Cos3 : Trigonometry
  Product{4..7} (4 alike) : Product
  Sum11 : Sum  Inputs=+-
  Sum12 : Sum
  alpha : Outport
  beta : Outport  Port=2
  wires:
  Cos3/1 -> Product6/2
  Product6/1 -> Sum12/1
  Sum11/1 -> alpha/1
  d/1 -> Product4/1, Product6/1
  wt/1 -> Cos3/1, Cos1/1, Cos2/1, Cos/1
  Product4/1 -> Sum11/1
  q/1 -> Product5/1, Product7/1
  Product7/1 -> Sum12/2
  Cos1/1 -> Product7/2
  Product5/1 -> Sum11/2
  Cos/1 -> Product4/2
  Cos2/1 -> Product5/2
  Sum12/1 -> beta/1

== system sim4el17128/wref/Signal Builder ==
  Demux : Demux  Tag=STV Demux  Outputs=3
  FromWs : FromWorkspace  Tag=STV FromWs  VariableName=tuvar  SampleTime=0
      SigBuilderData=|
      | common.afterFinalStr = 'Extrapolate'
      | common.sampleTime = 0
      | dataSet.timeRange = [0 25]
      | dataSet.name = 'Step wref'
      | sbobj.Groups.Name = 'Step wref'
      | sbobj.Groups.Signals(1).Name = 'wref'
      | sbobj.Groups.Signals(1).XData = [0 7 7 20 20 25]
      | sbobj.Groups.Signals(1).YData = [150 150 302.4 302.4 100 100]
      | sbobj.Groups.Signals(2).Name = 'wrefnom'
      | sbobj.Groups.Signals(2).XData = [0 25]
      | sbobj.Groups.Signals(2).YData = [150 150]
      | sbobj.Groups.Signals(3).Name = 'field weakening'
      | sbobj.Groups.Signals(3).XData = [0 25]
      | sbobj.Groups.Signals(3).YData = [1209.6 1209.6]
      | sbobj.Groups.TimeRange = [0 25]
  wref : Outport  Tag=STV Outport
  wrefnom : Outport  Tag=STV Outport  Port=2
  field weakening : Outport  Tag=STV Outport  Port=3
  wires:
  Demux/1 -> wref/1
  FromWs/1 -> Demux/1
  Demux/2 -> wrefnom/1
  Demux/3 -> field weakening/1

== system sim4el17128/Voltage Suply/Grid Voltage/abc to alphabeta ==
  a : Inport
  b : Inport  Port=2
  c : Inport  Port=3
  Gain2 : Gain  Gain=2/3
  Gain3 : Gain  Gain=1/3
  Gain4 : Gain  Gain=1/3
  Gain5 : Gain  Gain=0
  Gain6 : Gain  Gain=1/sqrt(3)
  Gain7 : Gain  Gain=1/sqrt(3)
  Sum : Sum  Inputs=+--
  Sum1 : Sum  Inputs=++-
  alpha : Outport
  beta : Outport  Port=2
  wires:
  Gain4/1 -> Sum/3
  Gain3/1 -> Sum/2
  a/1 -> Gain5/1, Gain2/1
  Gain6/1 -> Sum1/2
  c/1 -> Gain7/1, Gain4/1
  Gain7/1 -> Sum1/3
  Gain5/1 -> Sum1/1
  Gain2/1 -> Sum/1
  b/1 -> Gain6/1, Gain3/1
  Sum/1 -> alpha/1
  Sum1/1 -> beta/1

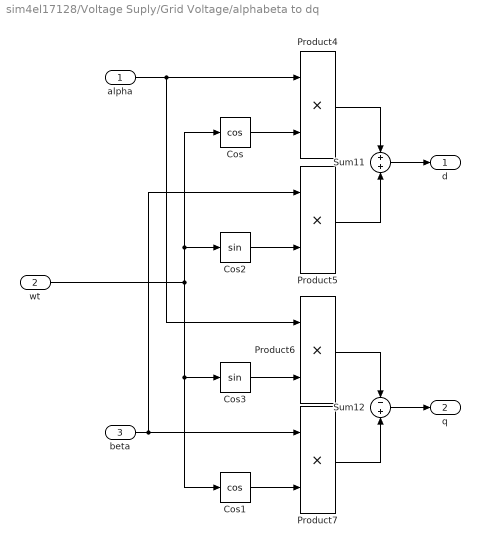
== system sim4el17128/Voltage Suply/Grid Voltage/alphabeta to dq ==
  alpha : Inport
  wt : Inport  Port=2
  beta : Inport  Port=3
  Cos : Trigonometry  Operator=cos
  Cos1 : Trigonometry  Operator=cos
  Cos2 : Trigonometry
  Cos3 : Trigonometry
  Product{4..7} (4 alike) : Product
  Sum11 : Sum
  Sum12 : Sum  Inputs=-+
  d : Outport
  q : Outport  Port=2
  wires:
  Cos3/1 -> Product6/2
  Product6/1 -> Sum12/1
  Sum11/1 -> d/1
  alpha/1 -> Product4/1, Product6/1
  wt/1 -> Cos3/1, Cos1/1, Cos2/1, Cos/1
  Product4/1 -> Sum11/1
  beta/1 -> Product5/1, Product7/1
  Product7/1 -> Sum12/2
  Cos1/1 -> Product7/2
  Product5/1 -> Sum11/2
  Cos/1 -> Product4/2
  Cos2/1 -> Product5/2
  Sum12/1 -> q/1
